simulink model "ex_9_sim"  (R2021a)
settings: Solver=FixedStepAuto  StartTime=0.0  StopTime=100  FixedStep=0.5  RelTol=1e-3
values from neighbouring files (symbols this model uses):
  a = [-1.6065;0.6065]    [ex_4.m]    (also in ex_5.m; ex_6_1.m = 1; ex_7.m; ex_8.m)
  am = [-1.3205;0.4966]    [ex_4.m]    (also in ex_5.m; ex_7.m; ex_8.m; ex_9_1.m)
  b = [0.1065;0.0902]    [ex_4.m]    (also in ex_5.m; ex_6_1.m = 1; ex_7.m; ex_8.m)
  bm = [0.1761;0]    [ex_4.m]    (also in ex_5.m = beta*b; ex_7.m; ex_8.m = beta*b; ex_9_1.m = beta*b)
  R1 = b(2)/b(1)    [ex_5_2.m]    (also in ex_7.m; ex_8.m = b(2)/b(1) + (b(2)^2-am(1)*b(1)*b(2)+am(2)*b(1)^2)*(-b(2)+a0*; ex_9_1.m = b(2)/b(1) + (b(2)^2-am(1)*b(1)*b(2)+am(2)*b(1)^2)*(-b(2)+a0*)
  S0 = (am(1)-a(1))/b(1)    [ex_5_2.m]    (also in ex_7.m; ex_8.m = b(2)*(a0*am(1)-a(2)-am(1)*a(1)+a(1)^2+am(2)-a(1)*a0)/(b(2)^2; ex_9_1.m = b(2)*(a0*am(1)-a(2)-am(1)*a(1)+a(1)^2+am(2)-a(1)*a0)/(b(2)^2)
  S1 = (am(2)-a(2))/b(1)    [ex_5_2.m]    (also in ex_7.m; ex_8.m = b(2)*(a(1)*a(2)-am(1)*a(2)+a0*am(2)-a0*a(2))/(b(2)^2-a(1)*b(; ex_9_1.m = b(2)*(a(1)*a(2)-am(1)*a(2)+a0*am(2)-a0*a(2))/(b(2)^2-a(1)*b()
settings Model: Creator=dbnun  LastModifiedBy=dimit

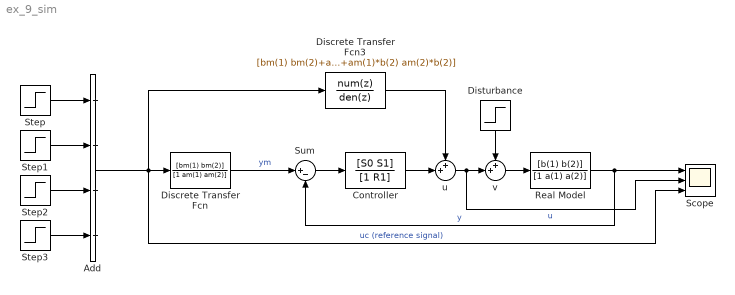
== system ex_9_sim ==
  Add : Sum  Inputs=++++
  Controller : DiscreteTransferFcn  Numerator=[S0 S1]  Denominator=[1 R1]
  Discrete Transfer Fcn : DiscreteTransferFcn  Numerator=[bm(1) bm(2)]  Denominator=[1 am(1) am(2)]  SampleTime=0.5
  Discrete Transfer Fcn3 : DiscreteTransferFcn  Numerator=[bm(1) bm(2)+a(1)*bm(1) a(1)*bm(2)+a(2)*bm(1) a(2)*bm(2)]  Denominator=[b(1) b(2)+b(1)*am(1) am(2)*b(1)+am(1)*b(2) am(2)*b(2)]
  Disturbance : Step  Time=40  After=0.5  SampleTime=0
  Real Model : DiscreteTransferFcn  Numerator=[b(1) b(2)]  Denominator=[1 a(1) a(2)]
  Scope : Scope  NumInputPorts=3
  Step : Step  Time=0  SampleTime=0
  Step1 : Step  Time=25  After=-2  SampleTime=0
  Step2 : Step  Time=50  After=2  SampleTime=0
  Step3 : Step  Time=75  After=-2  SampleTime=0
  Sum : Sum  Inputs=|+-
  u : Sum  Inputs=++|
  v : Sum  Inputs=++|
  wires:
  Step2/1 -> Add/3
  Step1/1 -> Add/2
  Add/1 -> Scope/3, Discrete Transfer Fcn3/1, Discrete Transfer Fcn/1  "uc (reference signal)"
  Step/1 -> Add/1
  Step3/1 -> Add/4
  Discrete Transfer Fcn/1 -> Sum/1  "ym"
  Sum/1 -> Controller/1
  Controller/1 -> u/2
  u/1 -> Scope/2, v/2  "u"
  Real Model/1 -> Scope/1, Sum/2  "y"
  Discrete Transfer Fcn3/1 -> u/1
  v/1 -> Real Model/1
  Disturbance/1 -> v/1
